simulink model "SAD_progetto"  (R2023b)
settings: Solver=ode4  StartTime=t0  StopTime=tf  FixedStep=t_step  RelTol=1e-3
model workspace (MAT data in the model file):
  N_order = 1
values from neighbouring files (symbols this model uses):
  A1 = importdata("igrfSg.txt")    [SAD_project_code.m]
  A2 = importdata("igrfSh.txt")    [SAD_project_code.m]
  A_1 = area_face(1)    [SAD_project_code.m]
  A_2 = area_face(2)    [SAD_project_code.m]
  A_3 = area_face(3)    [SAD_project_code.m]
  A_4 = area_face(4)    [SAD_project_code.m]
  A_5 = area_face(5)    [SAD_project_code.m]
  A_6 = area_face(6)    [SAD_project_code.m]
  alpha = [0.2 0.8]    [SAD_project_code.m]
  ARW = ARW*[1 1 1]'    [SAD_project_code.m]
  bias = bias*[1 1 1]'    [SAD_project_code.m]
  DCM_eci_per = rotationMatrix(rad2deg(i),rad2deg(OM), rad2deg(om))    [SAD_project_code.m]
  e = 0.0011241    [SAD_project_code.m]
  FS = 50000e-9    (= 5e-05)    [SAD_project_code.m]
  H0 = [g_10 g_11 h_11]'    [SAD_project_code.m]
  h_r_0 = [0,0,0]'    [SAD_project_code.m]
  horizon_cone_limit = deg2rad(70)    [SAD_project_code.m]
  I = 5/12.*diag([Ix Iy Iz])    [SAD_project_code.m]
  i = deg2rad(97.55)    [SAD_project_code.m]
  I_inv = inv(I)    [SAD_project_code.m]
  I_RW = 10    [SAD_project_code.m]
  I_vector_RW = [I_RW I_RW I_RW]'    [SAD_project_code.m]
  inc_tot = sqrt(inc_lin^2 + inc_acc^2)    [SAD_project_code.m]
  InitialTrueAnomalyOfEarth = 0    [SAD_project_code.m]
  j_b = [0.001 0.005 0.001]'    [SAD_project_code.m]
  matrix_RW_config = eye(3)    [SAD_project_code.m]
  matrix_RW_config_inv = inv(matrix_RW_config)    [SAD_project_code.m]
  mu_E = astroConstants(13)    [SAD_project_code.m]
  N_1 = BODY(1,:)    [SAD_project_code.m]
  N_2 = BODY(2,:)    [SAD_project_code.m]
  N_3 = BODY(3,:)    [SAD_project_code.m]
  N_4 = BODY(4,:)    [SAD_project_code.m]
  N_5 = BODY(5,:)    [SAD_project_code.m]
  N_6 = BODY(6,:)    [SAD_project_code.m]
  n_e = sqrt(mu_E/a^3)    [SAD_project_code.m]
  om = deg2rad(206.3209)    [SAD_project_code.m]
  OM = deg2rad(50.7464)    [SAD_project_code.m]
  p = a*(1-e^2)    [SAD_project_code.m]
  q0 = [0.1, -0.7, 0.51, 0.41]    [SAD_project_code.m]
  r_1 = r(1,:)    [SAD_project_code.m]
  r_2 = r(2,:)    [SAD_project_code.m]
  r_3 = r(3,:)    [SAD_project_code.m]
  r_4 = r(4,:)    [SAD_project_code.m]
  r_5 = r(5,:)    [SAD_project_code.m]
  r_6 = r(6,:)    [SAD_project_code.m]
  R_E = astroConstants(23)    [SAD_project_code.m]
  rho_d1 = 0.1    [SAD_project_code.m]
  rho_d2 = 0.1    [SAD_project_code.m]
  rho_d3 = 0.1    [SAD_project_code.m]
  rho_d4 = 0.1    [SAD_project_code.m]
  rho_d5 = 0.1    [SAD_project_code.m]
  rho_d6 = 0.1    [SAD_project_code.m]
  rho_s1 = rho_s(1)    [SAD_project_code.m]
  rho_s2 = rho_s(2)    [SAD_project_code.m]
  rho_s3 = rho_s(3)    [SAD_project_code.m]
  rho_s4 = rho_s(4)    [SAD_project_code.m]
  rho_s5 = rho_s(5)    [SAD_project_code.m]
  rho_s6 = rho_s(6)    [SAD_project_code.m]
  t_step = 0.01    [SAD_project_code.m]
  th0 = deg2rad(0)    [SAD_project_code.m]
  timeoflaunch = date2mjd2000(date0)    [SAD_project_code.m]
  ts_sensor = t_step*10    (= 0.1)    [SAD_project_code.m]
  w0 = [wx0 wy0 wz0]'    [SAD_project_code.m]
  w0_RW = [0 0 0]    [SAD_project_code.m]
  w_E = deg2rad(15.04)/60/60    [SAD_project_code.m]
  wMax_RW = 2*pi * RPM_max_RW / 60    (= 527.263967027)    [SAD_project_code.m]
libraries: matrix_library x41, dspindex x6, simulink x5, simulink_extras x4, aerolibutil x2, vrlib x2, dspinverses x1, slpidlib x1
(part 3 of 4)

== system SAD_progetto/Attitude determination and sensoring/Horizon Sensor/Normalize Vector1/Normalize Vector ==
  Vector : Inport
  Dot Product : DotProduct  OutDataTypeStr=Inherit: Inherit via internal rule
  Sqrt : Sqrt
  Norm : Outport
  wires:
  Sqrt/1 -> Norm/1
  Vector/1 -> Dot Product/1, Dot Product/2
  Dot Product/1 -> Sqrt/1

== system SAD_progetto/Attitude determination and sensoring/Horizon Sensor/Normalize Vector2/Normalize Vector ==
  Vector : Inport
  Dot Product : DotProduct  OutDataTypeStr=Inherit: Inherit via internal rule
  Sqrt : Sqrt
  Norm : Outport
  wires:
  Sqrt/1 -> Norm/1
  Vector/1 -> Dot Product/1, Dot Product/2
  Dot Product/1 -> Sqrt/1

== system SAD_progetto/Attitude determination and sensoring/Horizon Sensor/True Roll and Pitch betwen nadir and -z_body/Normalize Vector1 ==
  Vector : Inport
  Divide : Product  Inputs=*/
  Normalize Vector : Subsystem  AncestorBlock=LibrarySAD5/Normalize Vector1
  Versor : Outport
  wires:
  Vector/1 -> Normalize Vector/1(Vector), Divide/1
  Divide/1 -> Versor/1
  Normalize Vector/1(Norm) -> Divide/2

== system SAD_progetto/Attitude determination and sensoring/Subsystem1/Switch Case Action Only-Magnetometer/Subsystem ==
  B_b sensor : Inport
  B_N : Inport  Port=2
  Omega True : Inport  Port=3
  Cross Product4 : matrix_library/Cross Product
  DCM to quaternion : Subsystem
  Divide : Product  Inputs=*/
  Gain3 : Gain  Gain=1/ts_sensor
  Matrix Multiply2 : Product  Multiplication=Matrix(*)
  Norm vector : Subsystem  AncestorBlock=LibrarySAD5/Normalize Vector1
  Normalize Vector1 : Subsystem
  Normalize Vector5 : Subsystem
  Scope : Scope
  Square : Math  Operator=square
  Subsystem : Subsystem
  Subsystem1 : Subsystem
  Subtract3 : Sum  Inputs=+-
  Unit Delay2 : UnitDelay  InitialCondition=[1,0,0]'  SampleTime=-1  HasFrameUpgradeWarning=on
  time derivative : Subsystem
  q (scalar last) : Outport
  wires:
  time derivative/1(B_b dot Versor) -> Norm vector/1(Vector), Unit Delay2/1, Cross Product4/1  "B_b dot"
  Unit Delay2/1 -> Cross Product4/2
  Norm vector/1(Norm) -> Square/1
  Cross Product4/1 -> Divide/1
  Square/1 -> Divide/2
  Divide/1 -> Gain3/1
  Matrix Multiply2/1 -> DCM to quaternion/1(DCM)
  Normalize Vector1/1(Versor) -> Subsystem/1(B_b versor)  "B_b versor"
  Subsystem/1(b_matrix) -> Matrix Multiply2/1
  Normalize Vector5/1(Versor) -> Subsystem1/1(B_N versor)
  Subsystem1/1(r_matrix) -> Matrix Multiply2/2
  B_N/1 -> Normalize Vector5/1(Vector)
  Subtract3/1 -> Scope/1
  Gain3/1 -> Subtract3/2
  Omega True/1 -> Subtract3/1
  B_b sensor/1 -> time derivative/1(B_b), Normalize Vector1/1(Vector)
  DCM to quaternion/1(q (scalar last)) -> q (scalar last)/1

== system SAD_progetto/Attitude determination and sensoring/Subsystem1/Switch Case Action Statisitcal Attitude/Create matrix to statistical method ==
  Sensor1 (body frame) : Inport
  Sensor2 (body frame) : Inport  Port=2
  Reference1 (Inertial frame) : Inport  Port=3
  Reference2 (Inertial frame) : Inport  Port=4
  Matrix Concatenate1 : Concatenate  Mode=Multidimensional array  ConcatenateDimension=2
  Matrix Concatenate2 : Concatenate  Mode=Multidimensional array  ConcatenateDimension=2
  Normalize Vector1 : Subsystem
  Normalize Vector2 : Subsystem
  Normalize Vector3 : Subsystem
  Normalize Vector4 : Subsystem
  S matrix (body) : Outport
  V matrix (inertia) : Outport  Port=2
  wires:
  Matrix Concatenate1/1 -> V matrix (inertia)/1
  Normalize Vector1/1(Versor) -> Matrix Concatenate2/1
  Normalize Vector2/1(Versor) -> Matrix Concatenate2/2
  Normalize Vector4/1(Versor) -> Matrix Concatenate1/2
  Normalize Vector3/1(Versor) -> Matrix Concatenate1/1
  Matrix Concatenate2/1 -> S matrix (body)/1
  Reference1 (Inertial frame)/1 -> Normalize Vector3/1(Vector)
  Reference2 (Inertial frame)/1 -> Normalize Vector4/1(Vector)
  Sensor1 (body frame)/1 -> Normalize Vector1/1(Vector)
  Sensor2 (body frame)/1 -> Normalize Vector2/1(Vector)

== system SAD_progetto/Attitude determination and sensoring/Subsystem1/Switch Case Action Statisitcal Attitude/Statistical methods attitude determination (quaternion  Wabha’s problem)  ==
  note: In questo blocco ci sono altri metodi per il calcolo di q
  note: BLOCCO DA SISTEMARE SCEGLIENDO UNA SOLUZIONE
  note: Resolve linear system:
      | (𝑆 − σI)𝑞 + zq_4 = 𝜆_(MAX)*𝑞
      | 𝑧'𝑞 + σ*q_4 = 𝜆_(MAX)*𝑞_4
      |
      | Calculate eigenvalue (in the theory we assumed that lambda_max = 1)
  note: 𝐾 = [ (𝑆 − σI), 𝑧
      | 𝑧 ' 𝜎 ]
  note: 𝑧 = [𝑏23 − 𝑏32 , b31 − 𝑏13 , b12 − 𝑏21] '
  alpha (weigh of sensor) : Inport
  s matrix : Inport  Port=2
  v matrix : Inport  Port=3
  Adjoint of 3x3 Matrix : aerolibutil/Adjoint of 3x3 Matrix
  Blocco da convertire in formato simulink. Ho trovato 3 soluzioni differenti al proble : MATLAB Function  TreatAsAtomicUnit=on
  For Iterator Subsystem to calculate B matrix : Subsystem  TreatAsAtomicUnit=on
  Gain : Gain  Gain=eye(3)
  Matrix Concatenate : Concatenate  Mode=Multidimensional array  ConcatenateDimension=2
  Matrix Concatenate1 : Concatenate  Mode=Multidimensional array
  Matrix trace : Subsystem
  Subtract : Sum  Inputs=+-
  Sum : Sum  Inputs=|++
  Transpose : Math  Operator=transpose
  Transpose2 : Math  Operator=transpose
  Vector Concatenate1 : Concatenate
  Vector z : Subsystem
  q in quaternion (scalar last) : Outport
  wires:
  Transpose/1 -> Sum/2
  For Iterator Subsystem to calculate B matrix/1(B matrix) -> Vector z/1(B), Matrix trace/1(Matrix), Transpose/1, Sum/1  "B matrix"
  Sum/1 -> Adjoint of 3x3 Matrix/1, Blocco da convertire in formato simulink. Ho trovato 3 soluzioni differenti al proble/2(S), Subtract/1  "matrix S"
  Gain/1 -> Subtract/2
  Matrix trace/1(trace) -> Vector Concatenate1/2, Gain/1  "sigma = tr(B)"
  Matrix Concatenate/1 -> Matrix Concatenate1/1
  Vector Concatenate1/1 -> Transpose2/1
  Vector z/1(z) -> Vector Concatenate1/1, Matrix Concatenate/2
  Transpose2/1 -> Matrix Concatenate1/2
  Subtract/1 -> Matrix Concatenate/1  "S - sigma*eye(3)"
  alpha (weigh of sensor)/1 -> For Iterator Subsystem to calculate B matrix/1(alpha)
  v matrix/1 -> For Iterator Subsystem to calculate B matrix/3(v matrix)
  s matrix/1 -> For Iterator Subsystem to calculate B matrix/2(s matrix)
  Blocco da convertire in formato simulink. Ho trovato 3 soluzioni differenti al proble/1(q) -> q in quaternion (scalar last)/1  "q in quaternion (scalar last)"
  Adjoint of 3x3 Matrix/1 -> Blocco da convertire in formato simulink. Ho trovato 3 soluzioni differenti al proble/3(Sadj)
  Matrix Concatenate1/1 -> Blocco da convertire in formato simulink. Ho trovato 3 soluzioni differenti al proble/1(K)  "K matrix"

== system SAD_progetto/Attitude determination and sensoring/Subsystem1/Switch Case Action Triad Case/DCM to quaternion ==
  DCM : Inport
  Constant : Constant
  Divide : Product  Inputs=*/
  Extract Diagonal : matrix_library/Extract Diagonal
      settings: LibrarySourceBlock=|
      | simulink/Matrix
      | Operations/Extract Diagonal
  Gain : Gain  Gain=0.5
  Gain1 : Gain  Gain=[0 0 0; 0 0 1; 0 -1 0]
  Gain2 : Gain  Gain=[0 0 -1; 0 0 0; 1 0 0]
  Gain3 : Gain  Gain=[0 1 0; -1 0 0; 0 0 0]
  Gain4 : Gain  Gain=[4;4;4]
  Normalize Vector1 : Subsystem
  Sqrt : Sqrt
  Sum : Sum  Inputs=|++
  Sum of Elements{,1..3} (4 alike) : Sum  Inputs=+
  Vector Concatenate : Concatenate  NumInputs=3
  Vector Concatenate1 : Concatenate
  q (scalar last) : Outport
  wires:
  Extract Diagonal/1 -> Sum of Elements/1
  Sum of Elements/1 -> Sum/1
  Constant/1 -> Sum/2
  Sqrt/1 -> Gain/1
  DCM/1 -> Gain1/1, Gain2/1, Gain3/1, Extract Diagonal/1
  Gain2/1 -> Sum of Elements1/1
  Sum of Elements1/1 -> Vector Concatenate/2
  Gain1/1 -> Sum of Elements2/1
  Sum of Elements2/1 -> Vector Concatenate/1
  Sum of Elements3/1 -> Vector Concatenate/3
  Gain3/1 -> Sum of Elements3/1
  Vector Concatenate/1 -> Divide/1
  Gain/1 -> Vector Concatenate1/2, Gain4/1
  Divide/1 -> Vector Concatenate1/1
  Vector Concatenate1/1 -> Normalize Vector1/1(Vector)
  Normalize Vector1/1(Versor) -> q (scalar last)/1
  Sum/1 -> Sqrt/1
  Gain4/1 -> Divide/2

== system SAD_progetto/Attitude determination and sensoring/Subsystem1/Switch Case Action Triad Case/TRIAD: Attitude determination algebric Method with 2 sensor ==
  note: 𝑉^(-1) = 𝑉';
      | 𝐴 = 𝑆𝑉^(-1) = 𝑆𝑉'
  note: 𝑣1 = 𝑎;
      | 𝑣2 = (𝑎 ∧ 𝑏)/|𝑎 ∧ 𝑏|;
      | 𝑣3 = 𝑎 ∧ 𝑣2
  note: S1 = 𝑝;
      | 𝑠2 = (𝑝 ∧ 𝑞)/(|𝑝 ∧ 𝑞|);
      | 𝑠3 = 𝑝 ∧ 𝑠2
  Sensor1 (body frame) : Inport
  Sensor2 (body frame) : Inport  Port=2
  Reference1 (Inertial frame) : Inport  Port=3
  Reference2 (Inertial frame) : Inport  Port=4
  Matrix Multiply : Product  Multiplication=Matrix(*)
  Normalize Vector1 : Subsystem
  Normalize Vector2 : Subsystem
  Normalize Vector3 : Subsystem
  Normalize Vector4 : Subsystem
  Subsystem : Subsystem
  Subsystem1 : Subsystem
  Transpose : Math  Operator=transpose
  DCM_B/N  Att Det : Outport
  wires:
  Sensor1 (body frame)/1 -> Normalize Vector2/1(Vector)  "q"
  Sensor2 (body frame)/1 -> Normalize Vector3/1(Vector)  "p"
  Subsystem/1("Matrix S Measurements ") -> Matrix Multiply/1  "Matrix S Measurements (body frame)"
  Normalize Vector2/1(Versor) -> Subsystem/1(versor p (body frame))
  Normalize Vector3/1(Versor) -> Subsystem/2(versor q (body frame))
  Reference2 (Inertial frame)/1 -> Normalize Vector4/1(Vector)  "b"
  Reference1 (Inertial frame)/1 -> Normalize Vector1/1(Vector)  "a"
  Subsystem1/1("Matrix V certain model ") -> Transpose/1  "Matrix V (inertial frame)"
  Normalize Vector4/1(Versor) -> Subsystem1/2(versor b (inertial))
  Matrix Multiply/1 -> DCM_B/N  Att Det/1  "DCM_B/N from attirude determination"
  Transpose/1 -> Matrix Multiply/2
  Normalize Vector1/1(Versor) -> Subsystem1/1(versor a (inertial))

== system SAD_progetto/Calculation of disturbance torque/Solar pressure on 6 faces/Solar pressure on 6 faces1/Norm of vector ==
  Vector : Inport
  Dot Product : DotProduct  OutDataTypeStr=Inherit: Inherit via internal rule
  Sqrt : Sqrt
  Norm : Outport
  wires:
  Sqrt/1 -> Norm/1
  Vector/1 -> Dot Product/1, Dot Product/2
  Dot Product/1 -> Sqrt/1

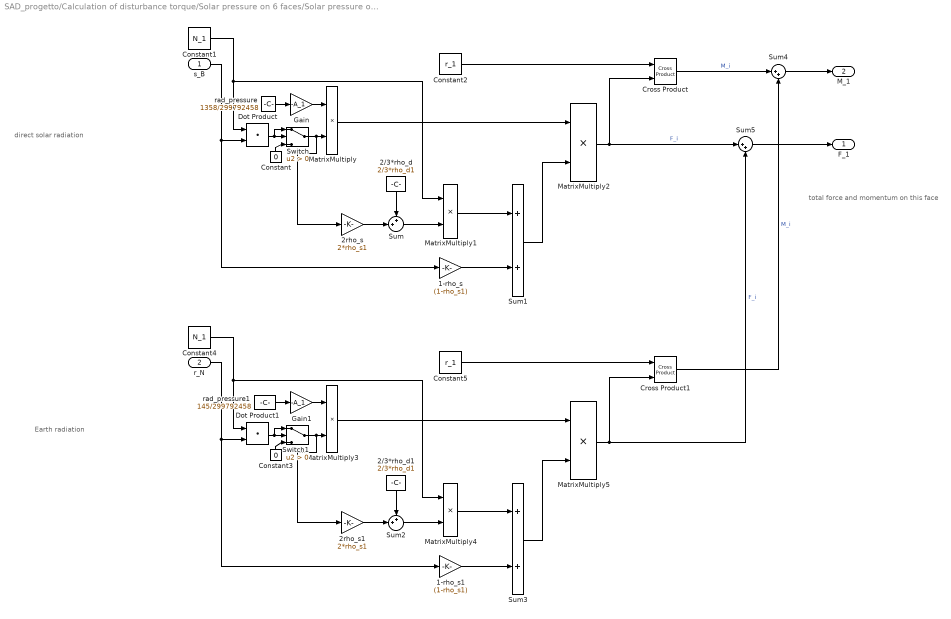
== system SAD_progetto/Calculation of disturbance torque/Solar pressure on 6 faces/Solar pressure on 6 faces1/solar pressure force and torque 1 ==
  note: total force and
      | momentum on this face
  note: direct solar radiation
  note: Earth radiation
  s_B : Inport
  r_N : Inport  Port=2
  1-rho_s : Gain  Gain=(1-rho_s1)
  1-rho_s1 : Gain  Gain=(1-rho_s1)
  2/3*rho_d : Constant  Value=2/3*rho_d1
  2/3*rho_d1 : Constant  Value=2/3*rho_d1
  2rho_s : Gain  Gain=2*rho_s1
  2rho_s1 : Gain  Gain=2*rho_s1
  Constant : Constant  Value=0
  Constant1 : Constant  Value=N_1
  Constant2 : Constant  Value=r_1
  Constant3 : Constant  Value=0
  Constant4 : Constant  Value=N_1
  Constant5 : Constant  Value=r_1
  Cross Product : matrix_library/Cross Product
  Cross Product1 : matrix_library/Cross Product
  Dot Product : DotProduct  OutDataTypeStr=Inherit: Inherit via internal rule
  Dot Product1 : DotProduct  OutDataTypeStr=Inherit: Inherit via internal rule
  Gain : Gain  Gain=-A_1
  Gain1 : Gain  Gain=-A_1
  MatrixMultiply{,1..5} (6 alike) : Product
  Sum : Sum  Inputs=++|
  Sum1 : Sum
  Sum2 : Sum  Inputs=++|
  Sum3 : Sum
  Sum4 : Sum  Inputs=|++
  Sum5 : Sum  Inputs=|++
  Switch : Switch  Criteria=u2 > Threshold  SaturateOnIntegerOverflow=off  InputSameDT=off
  Switch1 : Switch  Criteria=u2 > Threshold  SaturateOnIntegerOverflow=off  InputSameDT=off
  rad_pressure : Constant  Value=1358/299792458
  rad_pressure1 : Constant  Value=145/299792458
  F_1 : Outport
  M_1 : Outport  Port=2
  wires:
  MatrixMultiply2/1 -> Sum5/1, Cross Product/2  "F_i"
  MatrixMultiply/1 -> MatrixMultiply2/1
  Sum1/1 -> MatrixMultiply2/2
  s_B/1 -> 1-rho_s/1, Dot Product/2
  1-rho_s/1 -> Sum1/2
  rad_pressure/1 -> Gain/1
  MatrixMultiply1/1 -> Sum1/1
  Constant1/1 -> MatrixMultiply1/1, Dot Product/1
  Gain/1 -> MatrixMultiply/1
  Constant2/1 -> Cross Product/1
  Dot Product/1 -> Switch/1, Switch/2
  Constant/1 -> Switch/3
  Switch/1 -> 2rho_s/1, MatrixMultiply/2
  2rho_s/1 -> Sum/2
  2/3*rho_d/1 -> Sum/1
  Sum/1 -> MatrixMultiply1/2
  Sum3/1 -> MatrixMultiply5/2
  r_N/1 -> 1-rho_s1/1, Dot Product1/2
  1-rho_s1/1 -> Sum3/2
  2rho_s1/1 -> Sum2/2
  Switch1/1 -> 2rho_s1/1, MatrixMultiply3/2
  MatrixMultiply4/1 -> Sum3/1
  Constant5/1 -> Cross Product1/1
  MatrixMultiply3/1 -> MatrixMultiply5/1
  rad_pressure1/1 -> Gain1/1
  Constant3/1 -> Switch1/3
  Constant4/1 -> MatrixMultiply4/1, Dot Product1/1
  MatrixMultiply5/1 -> Sum5/2, Cross Product1/2  "F_i"
  Dot Product1/1 -> Switch1/1, Switch1/2
  Cross Product1/1 -> Sum4/2  "M_i"
  Sum2/1 -> MatrixMultiply4/2
  Gain1/1 -> MatrixMultiply3/1
  2/3*rho_d1/1 -> Sum2/1
  Sum4/1 -> M_1/1
  Cross Product/1 -> Sum4/1  "M_i"
  Sum5/1 -> F_1/1

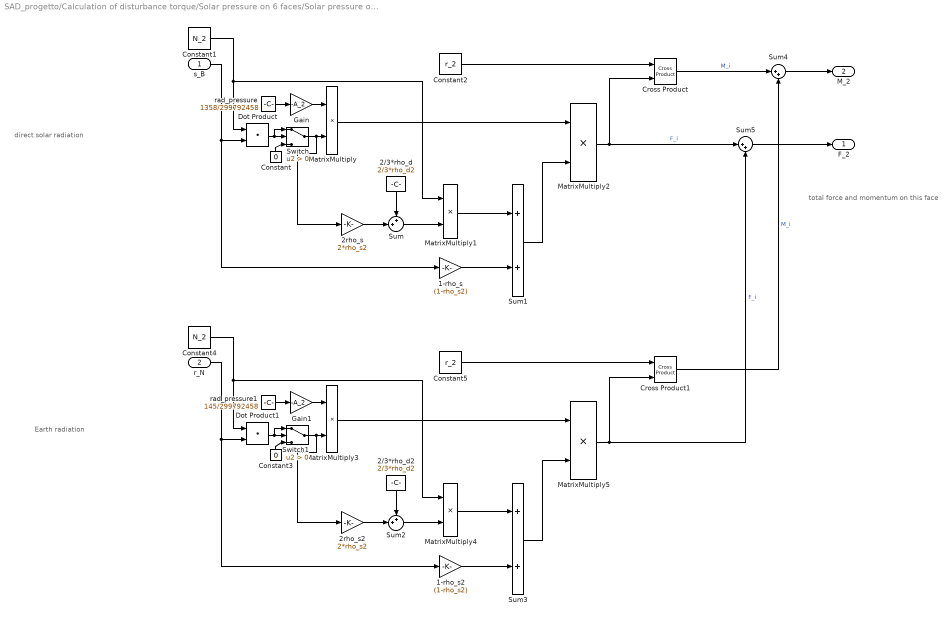
== system SAD_progetto/Calculation of disturbance torque/Solar pressure on 6 faces/Solar pressure on 6 faces1/solar pressure force and torque 2 ==
  note: total force and
      | momentum on this face
  note: direct solar radiation
  note: Earth radiation
  s_B : Inport
  r_N : Inport  Port=2
  1-rho_s : Gain  Gain=(1-rho_s2)
  1-rho_s2 : Gain  Gain=(1-rho_s2)
  2/3*rho_d : Constant  Value=2/3*rho_d2
  2/3*rho_d2 : Constant  Value=2/3*rho_d2
  2rho_s : Gain  Gain=2*rho_s2
  2rho_s2 : Gain  Gain=2*rho_s2
  Constant : Constant  Value=0
  Constant1 : Constant  Value=N_2
  Constant2 : Constant  Value=r_2
  Constant3 : Constant  Value=0
  Constant4 : Constant  Value=N_2
  Constant5 : Constant  Value=r_2
  Cross Product : matrix_library/Cross Product
  Cross Product1 : matrix_library/Cross Product
  Dot Product : DotProduct  OutDataTypeStr=Inherit: Inherit via internal rule
  Dot Product1 : DotProduct  OutDataTypeStr=Inherit: Inherit via internal rule
  Gain : Gain  Gain=-A_2
  Gain1 : Gain  Gain=-A_2
  MatrixMultiply{,1..5} (6 alike) : Product
  Sum : Sum  Inputs=++|
  Sum1 : Sum
  Sum2 : Sum  Inputs=++|
  Sum3 : Sum
  Sum4 : Sum  Inputs=|++
  Sum5 : Sum  Inputs=|++
  Switch : Switch  Criteria=u2 > Threshold  SaturateOnIntegerOverflow=off  InputSameDT=off
  Switch1 : Switch  Criteria=u2 > Threshold  SaturateOnIntegerOverflow=off  InputSameDT=off
  rad_pressure : Constant  Value=1358/299792458
  rad_pressure1 : Constant  Value=145/299792458
  F_2 : Outport
  M_2 : Outport  Port=2
  wires:
  MatrixMultiply2/1 -> Sum5/1, Cross Product/2  "F_i"
  MatrixMultiply/1 -> MatrixMultiply2/1
  Sum1/1 -> MatrixMultiply2/2
  s_B/1 -> 1-rho_s/1, Dot Product/2
  1-rho_s/1 -> Sum1/2
  rad_pressure/1 -> Gain/1
  MatrixMultiply1/1 -> Sum1/1
  Constant1/1 -> MatrixMultiply1/1, Dot Product/1
  Gain/1 -> MatrixMultiply/1
  Constant2/1 -> Cross Product/1
  Dot Product/1 -> Switch/1, Switch/2
  Constant/1 -> Switch/3
  Switch/1 -> 2rho_s/1, MatrixMultiply/2
  2rho_s/1 -> Sum/2
  2/3*rho_d/1 -> Sum/1
  Sum/1 -> MatrixMultiply1/2
  Sum3/1 -> MatrixMultiply5/2
  r_N/1 -> 1-rho_s2/1, Dot Product1/2
  1-rho_s2/1 -> Sum3/2
  2rho_s2/1 -> Sum2/2
  Switch1/1 -> 2rho_s2/1, MatrixMultiply3/2
  MatrixMultiply4/1 -> Sum3/1
  Constant5/1 -> Cross Product1/1
  MatrixMultiply3/1 -> MatrixMultiply5/1
  rad_pressure1/1 -> Gain1/1
  Constant3/1 -> Switch1/3
  Constant4/1 -> MatrixMultiply4/1, Dot Product1/1
  MatrixMultiply5/1 -> Sum5/2, Cross Product1/2  "F_i"
  Dot Product1/1 -> Switch1/1, Switch1/2
  Cross Product1/1 -> Sum4/2  "M_i"
  Sum2/1 -> MatrixMultiply4/2
  Gain1/1 -> MatrixMultiply3/1
  2/3*rho_d2/1 -> Sum2/1
  Sum4/1 -> M_2/1
  Cross Product/1 -> Sum4/1  "M_i"
  Sum5/1 -> F_2/1

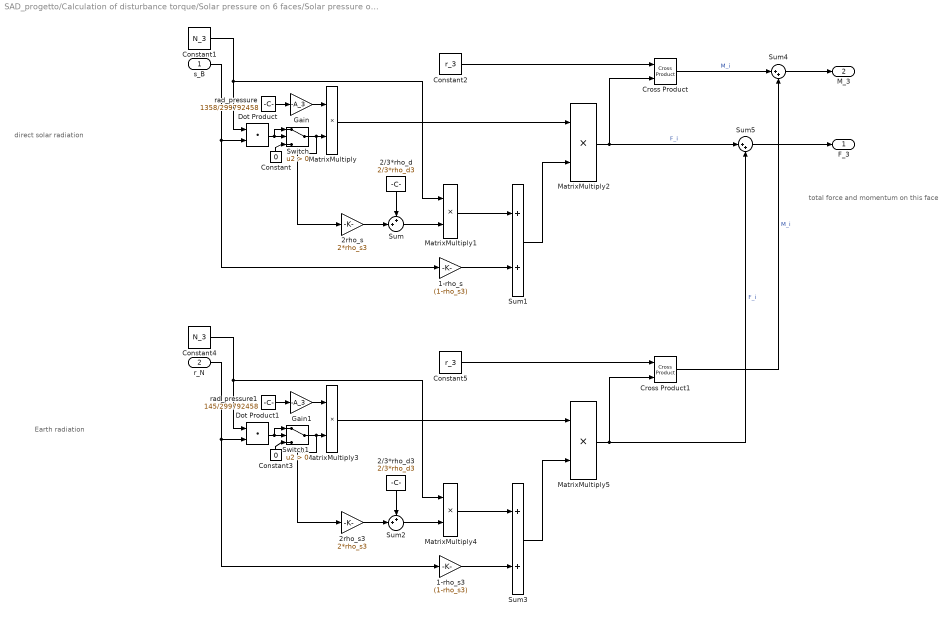
== system SAD_progetto/Calculation of disturbance torque/Solar pressure on 6 faces/Solar pressure on 6 faces1/solar pressure force and torque 3 ==
  note: total force and
      | momentum on this face
  note: direct solar radiation
  note: Earth radiation
  s_B : Inport
  r_N : Inport  Port=2
  1-rho_s : Gain  Gain=(1-rho_s3)
  1-rho_s3 : Gain  Gain=(1-rho_s3)
  2/3*rho_d : Constant  Value=2/3*rho_d3
  2/3*rho_d3 : Constant  Value=2/3*rho_d3
  2rho_s : Gain  Gain=2*rho_s3
  2rho_s3 : Gain  Gain=2*rho_s3
  Constant : Constant  Value=0
  Constant1 : Constant  Value=N_3
  Constant2 : Constant  Value=r_3
  Constant3 : Constant  Value=0
  Constant4 : Constant  Value=N_3
  Constant5 : Constant  Value=r_3
  Cross Product : matrix_library/Cross Product
  Cross Product1 : matrix_library/Cross Product
  Dot Product : DotProduct  OutDataTypeStr=Inherit: Inherit via internal rule
  Dot Product1 : DotProduct  OutDataTypeStr=Inherit: Inherit via internal rule
  Gain : Gain  Gain=-A_3
  Gain1 : Gain  Gain=-A_3
  MatrixMultiply{,1..5} (6 alike) : Product
  Sum : Sum  Inputs=++|
  Sum1 : Sum
  Sum2 : Sum  Inputs=++|
  Sum3 : Sum
  Sum4 : Sum  Inputs=|++
  Sum5 : Sum  Inputs=|++
  Switch : Switch  Criteria=u2 > Threshold  SaturateOnIntegerOverflow=off  InputSameDT=off
  Switch1 : Switch  Criteria=u2 > Threshold  SaturateOnIntegerOverflow=off  InputSameDT=off
  rad_pressure : Constant  Value=1358/299792458
  rad_pressure1 : Constant  Value=145/299792458
  F_3 : Outport
  M_3 : Outport  Port=2
  wires:
  MatrixMultiply2/1 -> Sum5/1, Cross Product/2  "F_i"
  MatrixMultiply/1 -> MatrixMultiply2/1
  Sum1/1 -> MatrixMultiply2/2
  s_B/1 -> 1-rho_s/1, Dot Product/2
  1-rho_s/1 -> Sum1/2
  rad_pressure/1 -> Gain/1
  MatrixMultiply1/1 -> Sum1/1
  Constant1/1 -> MatrixMultiply1/1, Dot Product/1
  Gain/1 -> MatrixMultiply/1
  Constant2/1 -> Cross Product/1
  Dot Product/1 -> Switch/1, Switch/2
  Constant/1 -> Switch/3
  Switch/1 -> 2rho_s/1, MatrixMultiply/2
  2rho_s/1 -> Sum/2
  2/3*rho_d/1 -> Sum/1
  Sum/1 -> MatrixMultiply1/2
  Sum3/1 -> MatrixMultiply5/2
  r_N/1 -> 1-rho_s3/1, Dot Product1/2
  1-rho_s3/1 -> Sum3/2
  2rho_s3/1 -> Sum2/2
  Switch1/1 -> 2rho_s3/1, MatrixMultiply3/2
  MatrixMultiply4/1 -> Sum3/1
  Constant5/1 -> Cross Product1/1
  MatrixMultiply3/1 -> MatrixMultiply5/1
  rad_pressure1/1 -> Gain1/1
  Constant3/1 -> Switch1/3
  Constant4/1 -> MatrixMultiply4/1, Dot Product1/1
  MatrixMultiply5/1 -> Sum5/2, Cross Product1/2  "F_i"
  Dot Product1/1 -> Switch1/1, Switch1/2
  Cross Product1/1 -> Sum4/2  "M_i"
  Sum2/1 -> MatrixMultiply4/2
  Gain1/1 -> MatrixMultiply3/1
  2/3*rho_d3/1 -> Sum2/1
  Sum4/1 -> M_3/1
  Cross Product/1 -> Sum4/1  "M_i"
  Sum5/1 -> F_3/1

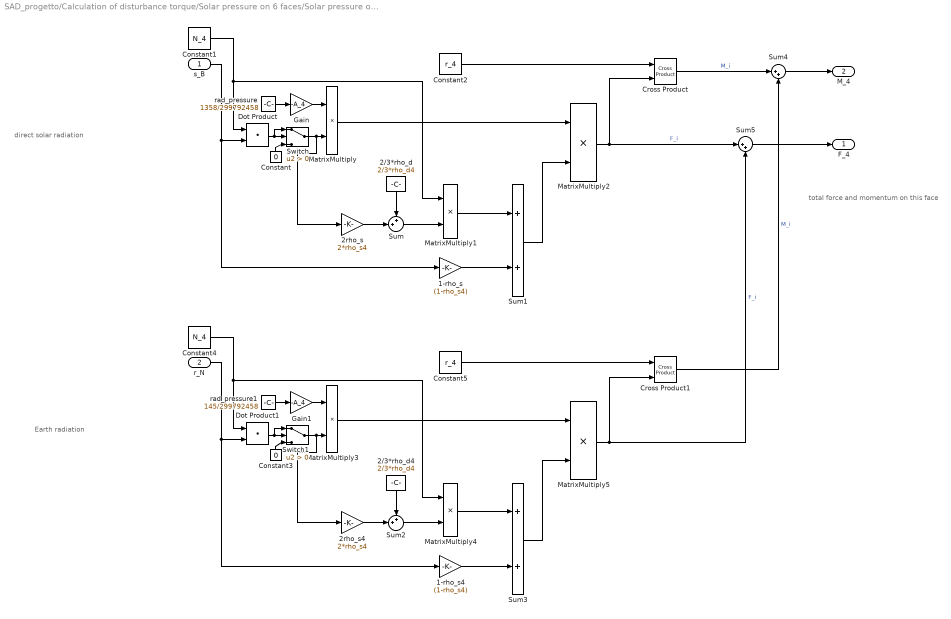
== system SAD_progetto/Calculation of disturbance torque/Solar pressure on 6 faces/Solar pressure on 6 faces1/solar pressure force and torque 4 ==
  note: total force and
      | momentum on this face
  note: direct solar radiation
  note: Earth radiation
  s_B : Inport
  r_N : Inport  Port=2
  1-rho_s : Gain  Gain=(1-rho_s4)
  1-rho_s4 : Gain  Gain=(1-rho_s4)
  2/3*rho_d : Constant  Value=2/3*rho_d4
  2/3*rho_d4 : Constant  Value=2/3*rho_d4
  2rho_s : Gain  Gain=2*rho_s4
  2rho_s4 : Gain  Gain=2*rho_s4
  Constant : Constant  Value=0
  Constant1 : Constant  Value=N_4
  Constant2 : Constant  Value=r_4
  Constant3 : Constant  Value=0
  Constant4 : Constant  Value=N_4
  Constant5 : Constant  Value=r_4
  Cross Product : matrix_library/Cross Product
  Cross Product1 : matrix_library/Cross Product
  Dot Product : DotProduct  OutDataTypeStr=Inherit: Inherit via internal rule
  Dot Product1 : DotProduct  OutDataTypeStr=Inherit: Inherit via internal rule
  Gain : Gain  Gain=-A_4
  Gain1 : Gain  Gain=-A_4
  MatrixMultiply{,1..5} (6 alike) : Product
  Sum : Sum  Inputs=++|
  Sum1 : Sum
  Sum2 : Sum  Inputs=++|
  Sum3 : Sum
  Sum4 : Sum  Inputs=|++
  Sum5 : Sum  Inputs=|++
  Switch : Switch  Criteria=u2 > Threshold  SaturateOnIntegerOverflow=off  InputSameDT=off
  Switch1 : Switch  Criteria=u2 > Threshold  SaturateOnIntegerOverflow=off  InputSameDT=off
  rad_pressure : Constant  Value=1358/299792458
  rad_pressure1 : Constant  Value=145/299792458
  F_4 : Outport
  M_4 : Outport  Port=2
  wires:
  MatrixMultiply2/1 -> Sum5/1, Cross Product/2  "F_i"
  MatrixMultiply/1 -> MatrixMultiply2/1
  Sum1/1 -> MatrixMultiply2/2
  s_B/1 -> 1-rho_s/1, Dot Product/2
  1-rho_s/1 -> Sum1/2
  rad_pressure/1 -> Gain/1
  MatrixMultiply1/1 -> Sum1/1
  Constant1/1 -> MatrixMultiply1/1, Dot Product/1
  Gain/1 -> MatrixMultiply/1
  Constant2/1 -> Cross Product/1
  Dot Product/1 -> Switch/1, Switch/2
  Constant/1 -> Switch/3
  Switch/1 -> 2rho_s/1, MatrixMultiply/2
  2rho_s/1 -> Sum/2
  2/3*rho_d/1 -> Sum/1
  Sum/1 -> MatrixMultiply1/2
  Sum3/1 -> MatrixMultiply5/2
  r_N/1 -> 1-rho_s4/1, Dot Product1/2
  1-rho_s4/1 -> Sum3/2
  2rho_s4/1 -> Sum2/2
  Switch1/1 -> 2rho_s4/1, MatrixMultiply3/2
  MatrixMultiply4/1 -> Sum3/1
  Constant5/1 -> Cross Product1/1
  MatrixMultiply3/1 -> MatrixMultiply5/1
  rad_pressure1/1 -> Gain1/1
  Constant3/1 -> Switch1/3
  Constant4/1 -> MatrixMultiply4/1, Dot Product1/1
  MatrixMultiply5/1 -> Sum5/2, Cross Product1/2  "F_i"
  Dot Product1/1 -> Switch1/1, Switch1/2
  Cross Product1/1 -> Sum4/2  "M_i"
  Sum2/1 -> MatrixMultiply4/2
  Gain1/1 -> MatrixMultiply3/1
  2/3*rho_d4/1 -> Sum2/1
  Sum4/1 -> M_4/1
  Cross Product/1 -> Sum4/1  "M_i"
  Sum5/1 -> F_4/1

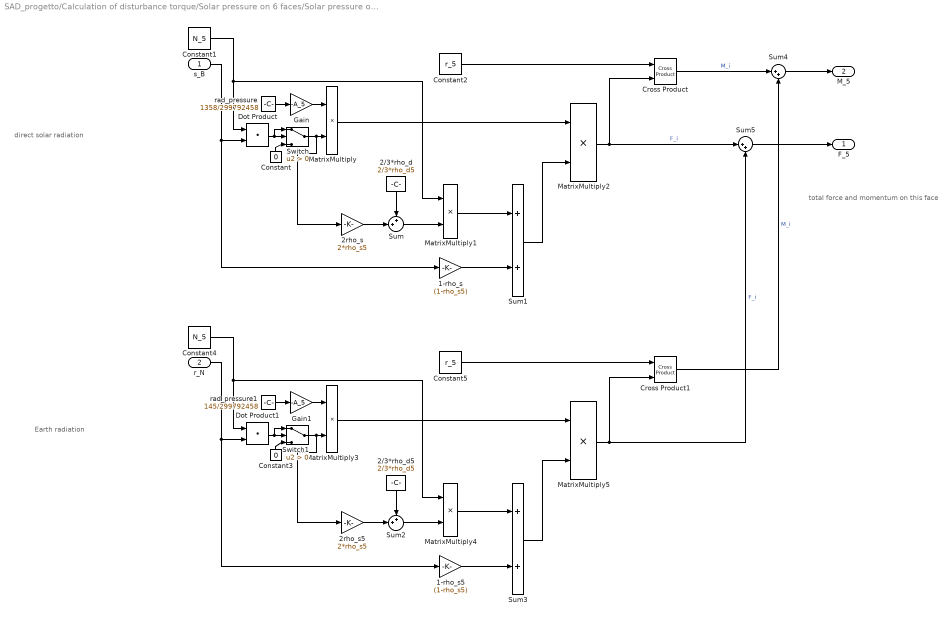
== system SAD_progetto/Calculation of disturbance torque/Solar pressure on 6 faces/Solar pressure on 6 faces1/solar pressure force and torque 5 ==
  note: total force and
      | momentum on this face
  note: direct solar radiation
  note: Earth radiation
  s_B : Inport
  r_N : Inport  Port=2
  1-rho_s : Gain  Gain=(1-rho_s5)
  1-rho_s5 : Gain  Gain=(1-rho_s5)
  2/3*rho_d : Constant  Value=2/3*rho_d5
  2/3*rho_d5 : Constant  Value=2/3*rho_d5
  2rho_s : Gain  Gain=2*rho_s5
  2rho_s5 : Gain  Gain=2*rho_s5
  Constant : Constant  Value=0
  Constant1 : Constant  Value=N_5
  Constant2 : Constant  Value=r_5
  Constant3 : Constant  Value=0
  Constant4 : Constant  Value=N_5
  Constant5 : Constant  Value=r_5
  Cross Product : matrix_library/Cross Product
  Cross Product1 : matrix_library/Cross Product
  Dot Product : DotProduct  OutDataTypeStr=Inherit: Inherit via internal rule
  Dot Product1 : DotProduct  OutDataTypeStr=Inherit: Inherit via internal rule
  Gain : Gain  Gain=-A_5
  Gain1 : Gain  Gain=-A_5
  MatrixMultiply{,1..5} (6 alike) : Product
  Sum : Sum  Inputs=++|
  Sum1 : Sum
  Sum2 : Sum  Inputs=++|
  Sum3 : Sum
  Sum4 : Sum  Inputs=|++
  Sum5 : Sum  Inputs=|++
  Switch : Switch  Criteria=u2 > Threshold  SaturateOnIntegerOverflow=off  InputSameDT=off
  Switch1 : Switch  Criteria=u2 > Threshold  SaturateOnIntegerOverflow=off  InputSameDT=off
  rad_pressure : Constant  Value=1358/299792458
  rad_pressure1 : Constant  Value=145/299792458
  F_5 : Outport
  M_5 : Outport  Port=2
  wires:
  MatrixMultiply2/1 -> Sum5/1, Cross Product/2  "F_i"
  MatrixMultiply/1 -> MatrixMultiply2/1
  Sum1/1 -> MatrixMultiply2/2
  s_B/1 -> 1-rho_s/1, Dot Product/2
  1-rho_s/1 -> Sum1/2
  rad_pressure/1 -> Gain/1
  MatrixMultiply1/1 -> Sum1/1
  Constant1/1 -> MatrixMultiply1/1, Dot Product/1
  Gain/1 -> MatrixMultiply/1
  Constant2/1 -> Cross Product/1
  Dot Product/1 -> Switch/1, Switch/2
  Constant/1 -> Switch/3
  Switch/1 -> 2rho_s/1, MatrixMultiply/2
  2rho_s/1 -> Sum/2
  2/3*rho_d/1 -> Sum/1
  Sum/1 -> MatrixMultiply1/2
  Sum3/1 -> MatrixMultiply5/2
  r_N/1 -> 1-rho_s5/1, Dot Product1/2
  1-rho_s5/1 -> Sum3/2
  2rho_s5/1 -> Sum2/2
  Switch1/1 -> 2rho_s5/1, MatrixMultiply3/2
  MatrixMultiply4/1 -> Sum3/1
  Constant5/1 -> Cross Product1/1
  MatrixMultiply3/1 -> MatrixMultiply5/1
  rad_pressure1/1 -> Gain1/1
  Constant3/1 -> Switch1/3
  Constant4/1 -> MatrixMultiply4/1, Dot Product1/1
  MatrixMultiply5/1 -> Sum5/2, Cross Product1/2  "F_i"
  Dot Product1/1 -> Switch1/1, Switch1/2
  Cross Product1/1 -> Sum4/2  "M_i"
  Sum2/1 -> MatrixMultiply4/2
  Gain1/1 -> MatrixMultiply3/1
  2/3*rho_d5/1 -> Sum2/1
  Sum4/1 -> M_5/1
  Cross Product/1 -> Sum4/1  "M_i"
  Sum5/1 -> F_5/1

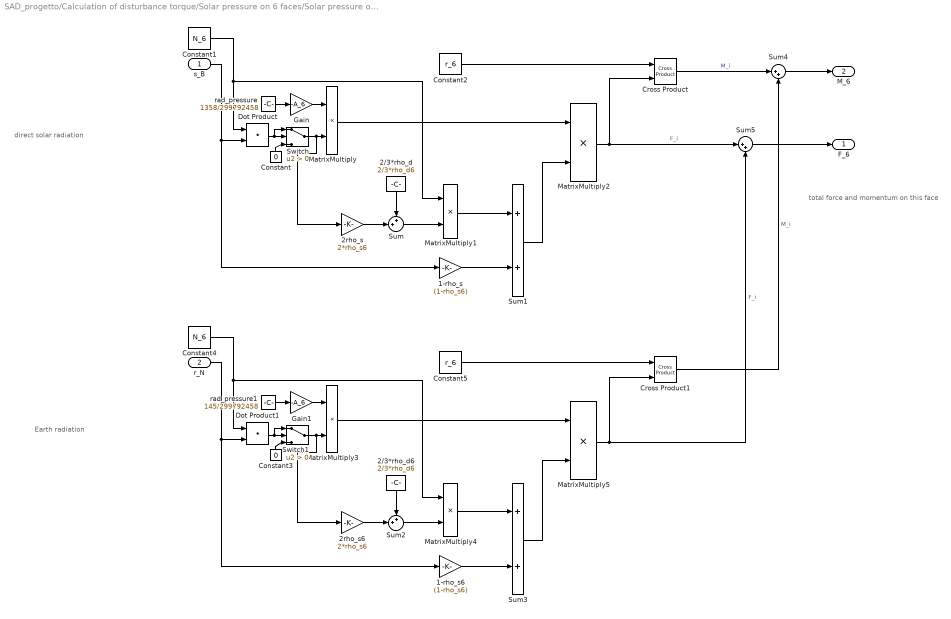
== system SAD_progetto/Calculation of disturbance torque/Solar pressure on 6 faces/Solar pressure on 6 faces1/solar pressure force and torque 6 ==
  note: total force and
      | momentum on this face
  note: direct solar radiation
  note: Earth radiation
  s_B : Inport
  r_N : Inport  Port=2
  1-rho_s : Gain  Gain=(1-rho_s6)
  1-rho_s6 : Gain  Gain=(1-rho_s6)
  2/3*rho_d : Constant  Value=2/3*rho_d6
  2/3*rho_d6 : Constant  Value=2/3*rho_d6
  2rho_s : Gain  Gain=2*rho_s6
  2rho_s6 : Gain  Gain=2*rho_s6
  Constant : Constant  Value=0
  Constant1 : Constant  Value=N_6
  Constant2 : Constant  Value=r_6
  Constant3 : Constant  Value=0
  Constant4 : Constant  Value=N_6
  Constant5 : Constant  Value=r_6
  Cross Product : matrix_library/Cross Product
  Cross Product1 : matrix_library/Cross Product
  Dot Product : DotProduct  OutDataTypeStr=Inherit: Inherit via internal rule
  Dot Product1 : DotProduct  OutDataTypeStr=Inherit: Inherit via internal rule
  Gain : Gain  Gain=-A_6
  Gain1 : Gain  Gain=-A_6
  MatrixMultiply{,1..5} (6 alike) : Product
  Sum : Sum  Inputs=++|
  Sum1 : Sum
  Sum2 : Sum  Inputs=++|
  Sum3 : Sum
  Sum4 : Sum  Inputs=|++
  Sum5 : Sum  Inputs=|++
  Switch : Switch  Criteria=u2 > Threshold  SaturateOnIntegerOverflow=off  InputSameDT=off
  Switch1 : Switch  Criteria=u2 > Threshold  SaturateOnIntegerOverflow=off  InputSameDT=off
  rad_pressure : Constant  Value=1358/299792458
  rad_pressure1 : Constant  Value=145/299792458
  F_6 : Outport
  M_6 : Outport  Port=2
  wires:
  MatrixMultiply2/1 -> Sum5/1, Cross Product/2  "F_i"
  MatrixMultiply/1 -> MatrixMultiply2/1
  Sum1/1 -> MatrixMultiply2/2
  s_B/1 -> 1-rho_s/1, Dot Product/2
  1-rho_s/1 -> Sum1/2
  rad_pressure/1 -> Gain/1
  MatrixMultiply1/1 -> Sum1/1
  Constant1/1 -> MatrixMultiply1/1, Dot Product/1
  Gain/1 -> MatrixMultiply/1
  Constant2/1 -> Cross Product/1
  Dot Product/1 -> Switch/1, Switch/2
  Constant/1 -> Switch/3
  Switch/1 -> 2rho_s/1, MatrixMultiply/2
  2rho_s/1 -> Sum/2
  2/3*rho_d/1 -> Sum/1
  Sum/1 -> MatrixMultiply1/2
  Sum3/1 -> MatrixMultiply5/2
  r_N/1 -> 1-rho_s6/1, Dot Product1/2
  1-rho_s6/1 -> Sum3/2
  2rho_s6/1 -> Sum2/2
  Switch1/1 -> 2rho_s6/1, MatrixMultiply3/2
  MatrixMultiply4/1 -> Sum3/1
  Constant5/1 -> Cross Product1/1
  MatrixMultiply3/1 -> MatrixMultiply5/1
  rad_pressure1/1 -> Gain1/1
  Constant3/1 -> Switch1/3
  Constant4/1 -> MatrixMultiply4/1, Dot Product1/1
  MatrixMultiply5/1 -> Sum5/2, Cross Product1/2  "F_i"
  Dot Product1/1 -> Switch1/1, Switch1/2
  Cross Product1/1 -> Sum4/2  "M_i"
  Sum2/1 -> MatrixMultiply4/2
  Gain1/1 -> MatrixMultiply3/1
  2/3*rho_d6/1 -> Sum2/1
  Sum4/1 -> M_6/1
  Cross Product/1 -> Sum4/1  "M_i"
  Sum5/1 -> F_6/1

== system SAD_progetto/Determine Control algorithm/Switch Case Action 3 axis stabilization Algorithm/DCM to quaternion/Normalize Vector1 ==
  Vector : Inport
  Divide : Product  Inputs=*/
  Norm vector : Subsystem  AncestorBlock=LibrarySAD5/Normalize Vector1
  Versor : Outport
  wires:
  Vector/1 -> Norm vector/1(Vector), Divide/1
  Divide/1 -> Versor/1
  Norm vector/1(Norm) -> Divide/2

== system SAD_progetto/Dynamics e Kinematics/Attitude error GG/calculating A_B//L/Subsystem ==
  note: A_L/N=A3(om+th)A1(i)A3(OM)
  Theta : Inport
  Constant : Constant  Value=[1,0,0;0 cos(i) sin(i); 0 -sin(i) cos(i)]
  Constant1 : Constant
  Constant2 : Constant  Value=0
  Constant3 : Constant  Value=om
  Constant4 : Constant  Value=[cos(OM),sin(OM),0;-sin(OM),cos(OM),0;0,0,1]
  Cos : Trigonometry  Operator=cos
  Gain : Gain  Gain=-1
  Matrix Concatenate : Concatenate  NumInputs=3  Mode=Multidimensional array  ConcatenateDimension=2
  Matrix Multiply : Product  Inputs=3  Multiplication=Matrix(*)
  Sin : Trigonometry
  Sum : Sum  Inputs=|++
  Vector Concatenate : Concatenate  NumInputs=3
  Vector Concatenate1 : Concatenate  NumInputs=3
  Vector Concatenate2 : Concatenate  NumInputs=3
  " A_L/N" : Outport
  wires:
  Vector Concatenate/1 -> Matrix Concatenate/1
  Vector Concatenate2/1 -> Matrix Concatenate/3
  Matrix Concatenate/1 -> Matrix Multiply/1
  Matrix Multiply/1 -> " A_L/N"/1
  Sin/1 -> Gain/1, Vector Concatenate1/1
  Gain/1 -> Vector Concatenate/2
  Vector Concatenate1/1 -> Matrix Concatenate/2
  Cos/1 -> Vector Concatenate/1, Vector Concatenate1/2
  Constant1/1 -> Vector Concatenate2/3
  Constant/1 -> Matrix Multiply/2
  Constant2/1 -> Vector Concatenate/3, Vector Concatenate1/3, Vector Concatenate2/1, Vector Concatenate2/2
  Theta/1 -> Sum/1
  Sum/1 -> Cos/1, Sin/1
  Constant3/1 -> Sum/2
  Constant4/1 -> Matrix Multiply/3

== system SAD_progetto/Enviroment Model/Magnetic Field/Switch Case Action Adavanced Magnetic model/Advanced magnetic field model ==
  note: INPUT:
      | - r_N are the coordinates of the satellite in the ECI frame
      | - A_bn is the DCM matrix to change from inertial frame to body frame
      | - timeoflaunch is the julian time at the start of simulation
      | - A1 and A2 are the matrices containing the coefficients of g and h up to the 13th order
      | - j_B is the residual magnetic induction
  note: the timeoflaunch is corrected by adding the time of simulation using a clock
  r_N : Inport
  N order : Inport  Port=2
  Clock1 : Clock
  Constant21 : Constant  Value=timeoflaunch
  Constant23 : Constant  Value=A1
  Constant24 : Constant  Value=A2
  Gain1 : Gain  Gain=1/(3600*24)
  MATLAB Function : MATLAB Function  TreatAsAtomicUnit=on
  Product3 : Product  Multiplication=Matrix(*)
  Rotation matrix for earth spin : Subsystem
  Sum : Sum  Inputs=|++
  cart to sph coord : Subsystem
  B_n : Outport
  wires:
  Rotation matrix for earth spin/1(eci_to_ecef) -> Product3/1
  Clock1/1 -> Gain1/1
  r_N/1 -> Product3/2
  Constant24/1 -> MATLAB Function/7(A2)
  cart to sph coord/3(long) -> MATLAB Function/4(LST), MATLAB Function/3(phi)
  Constant23/1 -> MATLAB Function/6(A1)
  Gain1/1 -> Sum/2
  Product3/1 -> cart to sph coord/1(r_xyz)
  cart to sph coord/2(lat) -> MATLAB Function/2(theta)
  Constant21/1 -> Sum/1
  Sum/1 -> MATLAB Function/5(mjd2000)
  cart to sph coord/1(r) -> MATLAB Function/1(r)
  MATLAB Function/1(B_n) -> B_n/1
  N order/1 -> MATLAB Function/8(N)

== system SAD_progetto/Enviroment Model/Magnetic Field/Switch Case Action Dipole model/Dipol Model of Magnetic Field ==
  note: CODE TO ADD
      | % Definition of Magnetic Field (Dipole model)
      |  j_b = [0.01 0.05 0.01]';
      | H0 = 1e-9.*[-29404.8 -1450.9 4652.5]';
  H0 vector : Inport
  EarthSat_n : Inport  Port=2
  Calculation of b_n : Subsystem
  b_N : Outport
  wires:
  H0 vector/1 -> Calculation of b_n/1(H0 vector)
  EarthSat_n/1 -> Calculation of b_n/2(EarthSat_n)
  Calculation of b_n/1(b_N) -> b_N/1

== system SAD_progetto/Enviroment Model/two-body Keplerian dynamics ECI/Integretion of true anomaly/(1-e^2)^(3//2) ==
  Constant1 : Constant
  Constant2 : Constant  Value=e
  Constant3 : Constant  Value=3/2
  Power : Math  Operator=pow
  Product1 : Product
  Subtract : Sum  Inputs=+-
  Out1 : Outport
  wires:
  Constant3/1 -> Power/2
  Constant2/1 -> Product1/2, Product1/1
  Subtract/1 -> Power/1
  Constant1/1 -> Subtract/1
  Product1/1 -> Subtract/2
  Power/1 -> Out1/1

== system SAD_progetto/Enviroment Model/two-body Keplerian dynamics ECI/r_perifocal/Calculation of norm r ==
  th : Inport
  Constant : Constant  Value=p
  Constant2 : Constant
  Cos : Trigonometry  Operator=cos
  Divide : Product  Inputs=*/
  Gain1 : Gain  Gain=e
  Sum : Sum  Inputs=|++
  Norm(r) : Outport
  wires:
  Constant/1 -> Divide/1
  Gain1/1 -> Sum/2
  Constant2/1 -> Sum/1
  Cos/1 -> Gain1/1
  Sum/1 -> Divide/2
  th/1 -> Cos/1
  Divide/1 -> Norm(r)/1

== system SAD_progetto/Subsystem/DCM to quaternion/Normalize Vector1/Norm vector ==
  Vector : Inport
  Dot Product : DotProduct  OutDataTypeStr=Inherit: Inherit via internal rule
  Sqrt : Sqrt
  Norm : Outport
  wires:
  Sqrt/1 -> Norm/1
  Vector/1 -> Dot Product/1, Dot Product/2
  Dot Product/1 -> Sqrt/1

== system SAD_progetto/Subsystem/Subsystem/Normalize Vector2/Norm vector ==
  Vector : Inport
  Dot Product : DotProduct  OutDataTypeStr=Inherit: Inherit via internal rule
  Sqrt : Sqrt
  Norm : Outport
  wires:
  Sqrt/1 -> Norm/1
  Vector/1 -> Dot Product/1, Dot Product/2
  Dot Product/1 -> Sqrt/1

== system SAD_progetto/Subsystem/Subsystem/Normalize Vector6/Norm vector ==
  Vector : Inport
  Dot Product : DotProduct  OutDataTypeStr=Inherit: Inherit via internal rule
  Sqrt : Sqrt
  Norm : Outport
  wires:
  Sqrt/1 -> Norm/1
  Vector/1 -> Dot Product/1, Dot Product/2
  Dot Product/1 -> Sqrt/1

== system SAD_progetto/Subsystem/Subsystem/time derivative/Normalize Vector2 ==
  Vector : Inport
  Divide : Product  Inputs=*/
  Norm vector : Subsystem  AncestorBlock=LibrarySAD5/Normalize Vector1
  Versor : Outport
  wires:
  Vector/1 -> Norm vector/1(Vector), Divide/1
  Divide/1 -> Versor/1
  Norm vector/1(Norm) -> Divide/2

== system SAD_progetto/Subsystem/Subsystem1/Normalize Vector2/Norm vector ==
  Vector : Inport
  Dot Product : DotProduct  OutDataTypeStr=Inherit: Inherit via internal rule
  Sqrt : Sqrt
  Norm : Outport
  wires:
  Sqrt/1 -> Norm/1
  Vector/1 -> Dot Product/1, Dot Product/2
  Dot Product/1 -> Sqrt/1

== system SAD_progetto/Subsystem/Subsystem1/Normalize Vector6/Norm vector ==
  Vector : Inport
  Dot Product : DotProduct  OutDataTypeStr=Inherit: Inherit via internal rule
  Sqrt : Sqrt
  Norm : Outport
  wires:
  Sqrt/1 -> Norm/1
  Vector/1 -> Dot Product/1, Dot Product/2
  Dot Product/1 -> Sqrt/1

== system SAD_progetto/Subsystem/Subsystem1/time derivative/Normalize Vector2 ==
  Vector : Inport
  Divide : Product  Inputs=*/
  Norm vector : Subsystem  AncestorBlock=LibrarySAD5/Normalize Vector1
  Versor : Outport
  wires:
  Vector/1 -> Norm vector/1(Vector), Divide/1
  Divide/1 -> Versor/1
  Norm vector/1(Norm) -> Divide/2

== system SAD_progetto/TRIAD: Attitude determination algebric Method with 2 sensor/Subsystem/Normalize Vector3/Normalize Vector ==
  Vector : Inport
  Dot Product : DotProduct  OutDataTypeStr=Inherit: Inherit via internal rule
  Sqrt : Sqrt
  Norm : Outport
  wires:
  Sqrt/1 -> Norm/1
  Vector/1 -> Dot Product/1, Dot Product/2
  Dot Product/1 -> Sqrt/1

== system SAD_progetto/TRIAD: Attitude determination algebric Method with 2 sensor/Subsystem1/Normalize Vector3/Normalize Vector ==
  Vector : Inport
  Dot Product : DotProduct  OutDataTypeStr=Inherit: Inherit via internal rule
  Sqrt : Sqrt
  Norm : Outport
  wires:
  Sqrt/1 -> Norm/1
  Vector/1 -> Dot Product/1, Dot Product/2
  Dot Product/1 -> Sqrt/1

== system SAD_progetto/Attitude determination and sensoring/Horizon Sensor/True Roll and Pitch betwen nadir and -z_body/Normalize Vector1/Normalize Vector ==
  Vector : Inport
  Dot Product : DotProduct  OutDataTypeStr=Inherit: Inherit via internal rule
  Sqrt : Sqrt
  Norm : Outport
  wires:
  Sqrt/1 -> Norm/1
  Vector/1 -> Dot Product/1, Dot Product/2
  Dot Product/1 -> Sqrt/1

== system SAD_progetto/Attitude determination and sensoring/Subsystem1/Switch Case Action Only-Magnetometer/Subsystem/DCM to quaternion ==
  DCM : Inport
  Abs : Abs  SaturateOnIntegerOverflow=off
  Constant : Constant
  Divide : Product  Inputs=*/
  Extract Diagonal : matrix_library/Extract Diagonal
      settings: LibrarySourceBlock=|
      | simulink/Matrix
      | Operations/Extract Diagonal
  Gain : Gain  Gain=0.5
  Gain1 : Gain  Gain=[0 0 0; 0 0 1; 0 -1 0]
  Gain2 : Gain  Gain=[0 0 -1; 0 0 0; 1 0 0]
  Gain3 : Gain  Gain=[0 1 0; -1 0 0; 0 0 0]
  Gain4 : Gain  Gain=[4;4;4]
  Normalize Vector1 : Subsystem
  Sqrt : Sqrt
  Sum : Sum  Inputs=|++
  Sum of Elements{,1..3} (4 alike) : Sum  Inputs=+
  Vector Concatenate : Concatenate  NumInputs=3
  Vector Concatenate1 : Concatenate
  q (scalar last) : Outport
  wires:
  Extract Diagonal/1 -> Sum of Elements/1
  Sum of Elements/1 -> Sum/1
  Constant/1 -> Sum/2
  Sqrt/1 -> Gain/1
  DCM/1 -> Gain1/1, Gain2/1, Gain3/1, Extract Diagonal/1
  Gain2/1 -> Sum of Elements1/1
  Sum of Elements1/1 -> Vector Concatenate/2
  Gain1/1 -> Sum of Elements2/1
  Sum of Elements2/1 -> Vector Concatenate/1
  Sum of Elements3/1 -> Vector Concatenate/3
  Gain3/1 -> Sum of Elements3/1
  Vector Concatenate/1 -> Divide/1
  Gain/1 -> Vector Concatenate1/2, Gain4/1
  Divide/1 -> Vector Concatenate1/1
  Vector Concatenate1/1 -> Normalize Vector1/1(Vector)
  Normalize Vector1/1(Versor) -> q (scalar last)/1
  Sum/1 -> Abs/1
  Gain4/1 -> Divide/2
  Abs/1 -> Sqrt/1

== system SAD_progetto/Attitude determination and sensoring/Subsystem1/Switch Case Action Only-Magnetometer/Subsystem/Norm vector ==
  Vector : Inport
  Dot Product : DotProduct  OutDataTypeStr=Inherit: Inherit via internal rule
  Sqrt : Sqrt
  Norm : Outport
  wires:
  Sqrt/1 -> Norm/1
  Vector/1 -> Dot Product/1, Dot Product/2
  Dot Product/1 -> Sqrt/1

== system SAD_progetto/Attitude determination and sensoring/Subsystem1/Switch Case Action Only-Magnetometer/Subsystem/Normalize Vector1 ==
  Vector : Inport
  Divide : Product  Inputs=*/
  Norm vector : Subsystem  AncestorBlock=LibrarySAD5/Normalize Vector1
  Versor : Outport
  wires:
  Vector/1 -> Norm vector/1(Vector), Divide/1
  Divide/1 -> Versor/1
  Norm vector/1(Norm) -> Divide/2

== system SAD_progetto/Attitude determination and sensoring/Subsystem1/Switch Case Action Only-Magnetometer/Subsystem/Normalize Vector5 ==
  Vector : Inport
  Divide : Product  Inputs=*/
  Norm vector : Subsystem  AncestorBlock=LibrarySAD5/Normalize Vector1
  Versor : Outport
  wires:
  Vector/1 -> Norm vector/1(Vector), Divide/1
  Divide/1 -> Versor/1
  Norm vector/1(Norm) -> Divide/2

== system SAD_progetto/Attitude determination and sensoring/Subsystem1/Switch Case Action Only-Magnetometer/Subsystem/Subsystem ==
  B_b versor : Inport
  Cross Product : matrix_library/Cross Product
  Cross Product1 : matrix_library/Cross Product
  Matrix Concatenate : Concatenate  NumInputs=3  Mode=Multidimensional array  ConcatenateDimension=2
  Matrix Multiply : Product  Multiplication=Matrix(*)
  Matrix Multiply1 : Product  Multiplication=Matrix(*)
  Normalize Vector1 : Subsystem
  Normalize Vector2 : Subsystem
  Normalize Vector6 : Subsystem
  Transpose : Math  Operator=transpose
  time derivative : Subsystem
  b_matrix : Outport
  wires:
  Matrix Multiply1/1 -> Normalize Vector1/1(Vector)  "b2 versor"
  B_b versor/1 -> Cross Product1/1, Matrix Concatenate/1, Matrix Multiply1/2, Cross Product/1, Matrix Multiply/1, time derivative/1(B_b versor)  "b1 versor"
  Transpose/1 -> Matrix Multiply/2
  Normalize Vector2/1(Versor) -> Matrix Concatenate/2, Cross Product1/2  "b3 versor"
  Matrix Multiply/1 -> Matrix Multiply1/1
  Cross Product/1 -> Normalize Vector2/1(Vector)
  Cross Product1/1 -> Normalize Vector6/1(Vector)
  Normalize Vector6/1(Versor) -> Matrix Concatenate/3  "b4 versor"
  Matrix Concatenate/1 -> b_matrix/1
  time derivative/1(B_b dot Versor) -> Transpose/1
  Normalize Vector1/1(Versor) -> Cross Product/2  "b3 versor"

== system SAD_progetto/Attitude determination and sensoring/Subsystem1/Switch Case Action Only-Magnetometer/Subsystem/Subsystem1 ==
  B_N versor : Inport
  Cross Product : matrix_library/Cross Product
  Cross Product1 : matrix_library/Cross Product
  Display : Display
  Display1 : Display
  Display2 : Display
  Matrix Concatenate : Concatenate  NumInputs=3  Mode=Multidimensional array  ConcatenateDimension=2
  Normalize Vector2 : Subsystem
  Normalize Vector6 : Subsystem
  time derivative : Subsystem
  r_matrix : Outport
  wires:
  time derivative/1(B_N dot Versor) -> Display/1, Cross Product/2  "r2 versor"
  B_N versor/1 -> Cross Product1/1, Matrix Concatenate/1, Display1/1, Cross Product/1, time derivative/1(B_N versor)  "r1 versor"
  Normalize Vector2/1(Versor) -> Matrix Concatenate/2, Cross Product1/2  "r3 versor"
  Cross Product/1 -> Display2/1, Normalize Vector2/1(Vector)
  Cross Product1/1 -> Normalize Vector6/1(Vector)
  Normalize Vector6/1(Versor) -> Matrix Concatenate/3  "r4 versor"
  Matrix Concatenate/1 -> r_matrix/1

== system SAD_progetto/Attitude determination and sensoring/Subsystem1/Switch Case Action Only-Magnetometer/Subsystem/time derivative ==
  B_b : Inport
  Gain1 : Gain  Gain=1/ ts_sensor
  Subtract : Sum  Inputs=+-
  Unit Delay : UnitDelay  InitialCondition=[0 0 0]'  SampleTime=-1  HasFrameUpgradeWarning=on
  B_b dot Versor : Outport
  wires:
  B_b/1 -> Subtract/1, Unit Delay/1
  Unit Delay/1 -> Subtract/2
  Subtract/1 -> Gain1/1  "B_b dot"
  Gain1/1 -> B_b dot Versor/1

== system SAD_progetto/Attitude determination and sensoring/Subsystem1/Switch Case Action Statisitcal Attitude/Create matrix to statistical method/Normalize Vector1 ==
  Vector : Inport
  Divide : Product  Inputs=*/
  Normalize Vector : Subsystem  AncestorBlock=LibrarySAD5/Normalize Vector1
  Versor : Outport
  wires:
  Vector/1 -> Normalize Vector/1(Vector), Divide/1
  Divide/1 -> Versor/1
  Normalize Vector/1(Norm) -> Divide/2

== system SAD_progetto/Attitude determination and sensoring/Subsystem1/Switch Case Action Statisitcal Attitude/Create matrix to statistical method/Normalize Vector2 ==
  Vector : Inport
  Divide : Product  Inputs=*/
  Normalize Vector : Subsystem  AncestorBlock=LibrarySAD5/Normalize Vector1
  Versor : Outport
  wires:
  Vector/1 -> Normalize Vector/1(Vector), Divide/1
  Divide/1 -> Versor/1
  Normalize Vector/1(Norm) -> Divide/2

== system SAD_progetto/Attitude determination and sensoring/Subsystem1/Switch Case Action Statisitcal Attitude/Create matrix to statistical method/Normalize Vector3 ==
  Vector : Inport
  Divide : Product  Inputs=*/
  Normalize Vector : Subsystem  AncestorBlock=LibrarySAD5/Normalize Vector1
  Versor : Outport
  wires:
  Vector/1 -> Normalize Vector/1(Vector), Divide/1
  Divide/1 -> Versor/1
  Normalize Vector/1(Norm) -> Divide/2

== system SAD_progetto/Attitude determination and sensoring/Subsystem1/Switch Case Action Statisitcal Attitude/Create matrix to statistical method/Normalize Vector4 ==
  Vector : Inport
  Divide : Product  Inputs=*/
  Normalize Vector : Subsystem  AncestorBlock=LibrarySAD5/Normalize Vector1
  Versor : Outport
  wires:
  Vector/1 -> Normalize Vector/1(Vector), Divide/1
  Divide/1 -> Versor/1
  Normalize Vector/1(Norm) -> Divide/2

== system SAD_progetto/Attitude determination and sensoring/Subsystem1/Switch Case Action Statisitcal Attitude/Statistical methods attitude determination (quaternion  Wabha’s problem) /For Iterator Subsystem to calculate B matrix ==
  note: Remember the last matrix B
  note: count the index
      | Important to flag reset in "State variable" to reset unit delay
  note: It's a for loop that resolve this expression
      | 𝐵 = ∑ 𝛼_𝑖*𝑠_𝑖*𝑣_𝑖' = [𝑏ij] to obatain matix B that it is a square matrix of order 3
      |
      | Analogous code for the iteration:
      |
      | for i = 1:size(alpha,2)
      | B = B + alpha(i)*s(:,i)*v(:,i)'
      | end
  alpha : Inport
  s matrix : Inport  Port=2
  v matrix : Inport  Port=3
  Add : Sum
  For Iterator : ForIterator  ResetStates=reset  IterationLimit=size(alpha,2)
  Matrix Multiply : Product  Multiplication=Matrix(*)
  Product : Product
  Transpose : Math  Operator=transpose
  Unit Delay1 : UnitDelay  SampleTime=-1  HasFrameUpgradeWarning=on
  Variable Selector : dspindex/Variable Selector  NumInputs=1  rowsOrCols=Columns  IdxMode=Variable  Elements=[1 3]  ZerOneIdxMode=One-based  errmode=Clip Index  FillMode=on  FillValues=0
  Variable Selector1 : dspindex/Variable Selector  NumInputs=1  rowsOrCols=Columns  IdxMode=Variable  Elements=[1 3]  ZerOneIdxMode=One-based  errmode=Clip Index  FillMode=on  FillValues=0
  Variable Selector2 : dspindex/Variable Selector  NumInputs=1  rowsOrCols=Columns  IdxMode=Variable  Elements=[1 3]  ZerOneIdxMode=One-based  errmode=Clip Index  FillMode=on  FillValues=0
  B matrix : Outport
  wires:
  For Iterator/1 -> Variable Selector1/2, Variable Selector/2, Variable Selector2/2
  alpha/1 -> Variable Selector2/1
  s matrix/1 -> Variable Selector/1
  Variable Selector2/1 -> Product/1
  Variable Selector/1 -> Product/2
  Product/1 -> Matrix Multiply/1
  Variable Selector1/1 -> Transpose/1
  Transpose/1 -> Matrix Multiply/2
  Matrix Multiply/1 -> Add/1
  v matrix/1 -> Variable Selector1/1
  Unit Delay1/1 -> Add/2
  Add/1 -> Unit Delay1/1, B matrix/1

== system SAD_progetto/Attitude determination and sensoring/Subsystem1/Switch Case Action Statisitcal Attitude/Statistical methods attitude determination (quaternion  Wabha’s problem) /Matrix trace ==
  Matrix : Inport
  Extract Diagonal : matrix_library/Extract Diagonal
      settings: LibrarySourceBlock=|
      | simulink/Matrix
      | Operations/Extract Diagonal
  Sum of Elements : Sum  Inputs=+
  trace : Outport
  wires:
  Extract Diagonal/1 -> Sum of Elements/1
  Sum of Elements/1 -> trace/1  "sigma"
  Matrix/1 -> Extract Diagonal/1

== system SAD_progetto/Attitude determination and sensoring/Subsystem1/Switch Case Action Statisitcal Attitude/Statistical methods attitude determination (quaternion  Wabha’s problem) /Vector z ==
  B : Inport
  Gain1 : Gain  Gain=-1
  Selector : Selector  NumberOfDimensions=2  InputPortWidth=3  IndexOptions=Index vector (dialog),Starting index (dialog)  Indices=2,3  OutputSizes=1,1
  Selector1 : Selector  NumberOfDimensions=2  InputPortWidth=3  IndexOptions=Index vector (dialog),Starting index (dialog)  Indices=1,3  OutputSizes=1,1
  Selector2 : Selector  NumberOfDimensions=2  InputPortWidth=3  IndexOptions=Index vector (dialog),Starting index (dialog)  Indices=1,2  OutputSizes=1,1
  Subtract1 : Sum  Inputs=+-
  Transpose1 : Math  Operator=transpose
  Vector Concatenate : Concatenate  NumInputs=3
  z : Outport
  wires:
  B/1 -> Subtract1/1, Transpose1/1
  Transpose1/1 -> Subtract1/2
  Selector2/1 -> Vector Concatenate/3
  Selector/1 -> Vector Concatenate/1
  Subtract1/1 -> Selector/1, Selector2/1, Selector1/1
  Vector Concatenate/1 -> z/1
  Gain1/1 -> Vector Concatenate/2
  Selector1/1 -> Gain1/1

== system SAD_progetto/Attitude determination and sensoring/Subsystem1/Switch Case Action Triad Case/DCM to quaternion/Normalize Vector1 ==
  Vector : Inport
  Divide : Product  Inputs=*/
  Norm vector : Subsystem  AncestorBlock=LibrarySAD5/Normalize Vector1
  Versor : Outport
  wires:
  Vector/1 -> Norm vector/1(Vector), Divide/1
  Divide/1 -> Versor/1
  Norm vector/1(Norm) -> Divide/2

== system SAD_progetto/Attitude determination and sensoring/Subsystem1/Switch Case Action Triad Case/TRIAD: Attitude determination algebric Method with 2 sensor/Normalize Vector1 ==
  Vector : Inport
  Divide : Product  Inputs=*/
  Normalize Vector : Subsystem  AncestorBlock=LibrarySAD5/Normalize Vector1
  Versor : Outport
  wires:
  Vector/1 -> Normalize Vector/1(Vector), Divide/1
  Divide/1 -> Versor/1
  Normalize Vector/1(Norm) -> Divide/2
